simulink model "newMotorModelSfn"  (R2019a)
settings: Solver=VariableStepAuto  StartTime=0.0  StopTime=12000  FixedStep=.0001  RelTol=1e-3
libraries: simulink x1
settings Model: Creator=tdarrah  LastModifiedBy=tdarrah

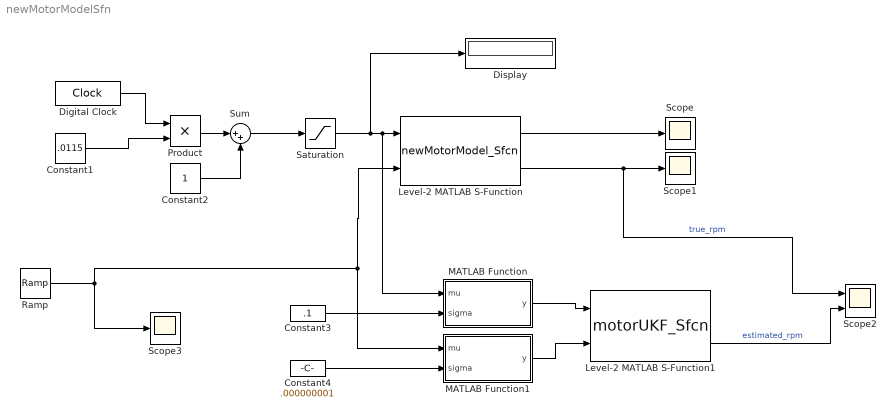
== system newMotorModelSfn ==
  Constant1 : Constant  Value=.0115
  Constant2 : Constant
  Constant3 : Constant  Value=.1
  Constant4 : Constant  Value=.000000001
  Digital Clock : DigitalClock
  Display : Display
  Level-2 MATLAB S-Function : M-S-Function  FunctionName=newMotorModel_Sfcn  Parameters=motorParams
      mask Display:
      | port_label('input', 1, 'voltage');
      | port_label('input', 2, 'friction');
      | port_label('output', 1, 'current');
      | port_label('output', 2, 'rpm');
      | disp("BLDC Motor");
  Level-2 MATLAB S-Function1 : M-S-Function  FunctionName=motorUKF_Sfcn  Parameters=motorParams
      mask Display:
      | port_label('input', 1, 'voltage');
      | port_label('input', 2, 'friction');
      | port_label('output', 1, 'current');
      | port_label('output', 2, 'rpm_hat');
      | disp("Motor UKF");
  MATLAB Function : MATLAB Function  TreatAsAtomicUnit=on
  MATLAB Function1 : MATLAB Function  TreatAsAtomicUnit=on
  Product : Product
  Ramp : simulink/Sources/Ramp  slope=.000000001  start=500000  InitialOutput=1.16e-4
  Saturation : Saturate  UpperLimit=11.4  LowerLimit=0
  Scope : Scope
  Scope1 : Scope
  Scope2 : Scope  NumInputPorts=2
  Scope3 : Scope
  Sum : Sum  Inputs=|++
  wires:
  Level-2 MATLAB S-Function/1 -> Scope/1
  Level-2 MATLAB S-Function/2 -> Scope2/1, Scope1/1  "true_rpm"
  Saturation/1 -> Display/1, MATLAB Function/1(mu), Level-2 MATLAB S-Function/1
  Product/1 -> Sum/1
  Digital Clock/1 -> Product/1
  Constant1/1 -> Product/2
  Constant2/1 -> Sum/2
  Sum/1 -> Saturation/1
  MATLAB Function/1(y) -> Level-2 MATLAB S-Function1/1
  MATLAB Function1/1(y) -> Level-2 MATLAB S-Function1/2
  Constant3/1 -> MATLAB Function/2(sigma)
  Constant4/1 -> MATLAB Function1/2(sigma)
  Level-2 MATLAB S-Function1/2 -> Scope2/2  "estimated_rpm"
  Ramp/1 -> Scope3/1, Level-2 MATLAB S-Function/2, MATLAB Function1/1(mu)

== matlab function newMotorModelSfn/MATLAB Function1 ==
  settings: updateMethod=DISCRETE  sampleTime=.2
  data: mu input; y output; sigma input
function y = addNoise(mu, sigma)

y = normrnd(mu, sigma);

== matlab function newMotorModelSfn/MATLAB Function ==
  settings: updateMethod=DISCRETE  sampleTime=.2
  data: mu input; y output; sigma input
function y = addNoise(mu, sigma)

y = normrnd(mu, sigma);
